simulink model "PF1_Q3"  (R2023b)
settings: Solver=FixedStepAuto  StartTime=0  StopTime=100  FixedStep=0.01  RelTol=1e-3
values from neighbouring files (symbols this model uses):
  B = double([diff(Xdot(1), u) ... (first row only)    [PF1.m]    (also in PF1_Q4.m)
  C = [1 0]    [PF1.m]    (also in PF1_Q4.m)
  K = place(A2, B, lambda_cl)    [PF1.m]    (also in PF1_Q4.m)
  K2 = place(A3, B, lambda_cl)    [PF1.m]    (also in PF1_Q4.m)
  Ki = -10    [PF1.m]    (also in PF1_Q4.m)
  xeq1 = double([eq.x1(1) ... (first row only)    [PF1.m]    (also in PF1_Q4.m = [0)
  xeq2 = double([eq.x1(2) ... (first row only)    [PF1.m]    (also in PF1_Q4.m = [1/2)
  xeq3 = [5 ... (first row only)    [PF1.m]    (also in PF1_Q4.m)
libraries: simulink x1
settings Model: Creator=therk  LastModifiedBy=Therkelsen

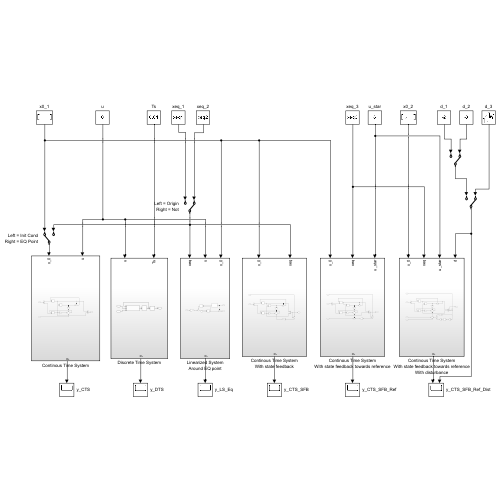
[thumbnail: Simulink's stored preview of the top-level diagram]
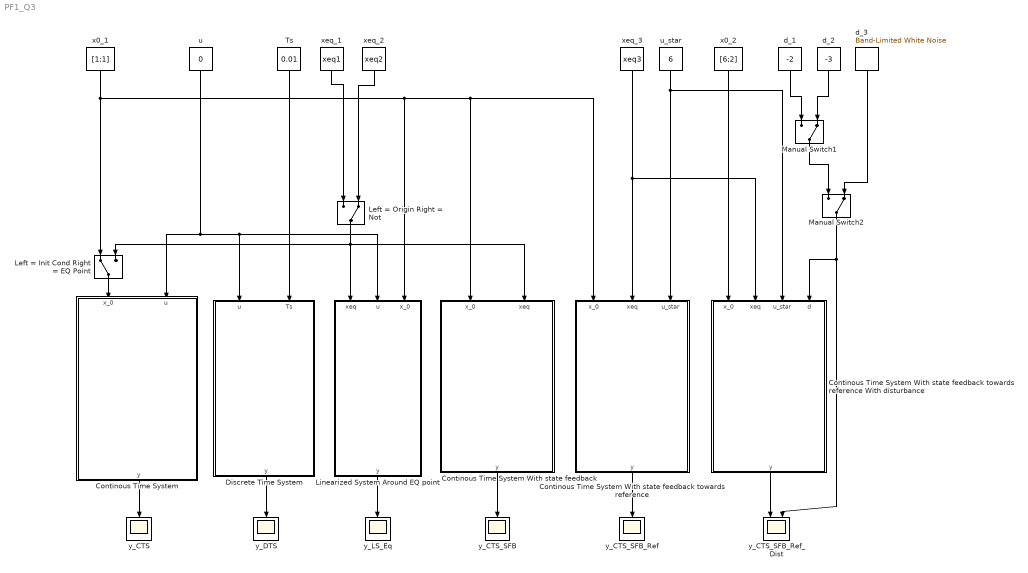
== system PF1_Q3 ==
  Continous Time System : Subsystem
  Continous Time System With state feedback : Subsystem
  Continous Time System With state feedback towards reference : Subsystem
  Continous Time System With state feedback towards reference With disturbance : Subsystem
  Discrete Time System : Subsystem
  Left = Init Cond Right = EQ Point : ManualSwitch
  Left = Origin Right = Not : ManualSwitch  CurrentSetting=0
  Linearized System Around EQ point : Subsystem
  Manual Switch1 : ManualSwitch  CurrentSetting=0
  Manual Switch2 : ManualSwitch  CurrentSetting=0
  Ts : Constant  Value=0.01
  d_1 : Constant  Value=-2
  d_2 : Constant  Value=-3
  d_3 : simulink/Sources/Band-Limited White Noise  Cov=[10]  Ts=10  seed=[23341]
  u : Constant  Value=0
  u_star : Constant  Value=6
  x0_1 : Constant  Value=[1;1]
  x0_2 : Constant  Value=[6;2]
  xeq_1 : Constant  Value=xeq1
  xeq_2 : Constant  Value=xeq2
  xeq_3 : Constant  Value=xeq3
  y_CTS : Scope
  y_CTS_SFB : Scope
  y_CTS_SFB_Ref : Scope
  y_CTS_SFB_Ref_Dist : Scope  NumInputPorts=2
  y_DTS : Scope
  y_LS_Eq : Scope
  wires:
  Continous Time System/1(y) -> y_CTS/1
  Ts/1 -> Discrete Time System/2(Ts)
  Discrete Time System/1(y) -> y_DTS/1
  xeq_2/1 -> Left = Origin Right = Not/2
  xeq_1/1 -> Left = Origin Right = Not/1
  Left = Origin Right = Not/1 -> Linearized System Around EQ point/1(xeq), Continous Time System With state feedback/2(xeq), Left = Init Cond Right = EQ Point/2
  u/1 -> Linearized System Around EQ point/2(u), Discrete Time System/1(u), Continous Time System/2(u)
  Linearized System Around EQ point/1(y) -> y_LS_Eq/1
  x0_1/1 -> Continous Time System With state feedback towards reference/1(x_0), Continous Time System With state feedback/1(x_0), Linearized System Around EQ point/3(x_0), Left = Init Cond Right = EQ Point/1
  Left = Init Cond Right = EQ Point/1 -> Continous Time System/1(x_0)
  Continous Time System With state feedback/1(y) -> y_CTS_SFB/1
  u_star/1 -> Continous Time System With state feedback towards reference With disturbance/3(u_star), Continous Time System With state feedback towards reference/3(u_star)
  Continous Time System With state feedback towards reference/1(y) -> y_CTS_SFB_Ref/1
  xeq_3/1 -> Continous Time System With state feedback towards reference With disturbance/2(xeq), Continous Time System With state feedback towards reference/2(xeq)
  Continous Time System With state feedback towards reference With disturbance/1(y) -> y_CTS_SFB_Ref_Dist/1
  d_1/1 -> Manual Switch1/1
  d_2/1 -> Manual Switch1/2
  x0_2/1 -> Continous Time System With state feedback towards reference With disturbance/1(x_0)
  d_3/1 -> Manual Switch2/2
  Manual Switch1/1 -> Manual Switch2/1
  Manual Switch2/1 -> y_CTS_SFB_Ref_Dist/2, Continous Time System With state feedback towards reference With disturbance/4(d)

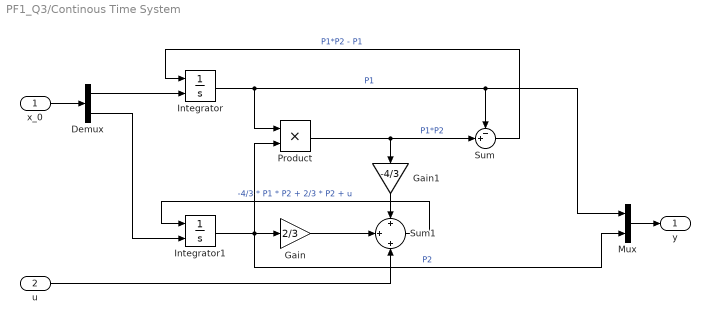
== system PF1_Q3/Continous Time System ==
  x_0 : Inport
  u : Inport  Port=2
  Demux : Demux  Outputs=2
  Gain : Gain  Gain=2/3
  Gain1 : Gain  Gain=-4/3
  Integrator : Integrator  InitialConditionSource=external
  Integrator1 : Integrator  InitialConditionSource=external
  Mux : Mux  Inputs=2
  Product : Product
  Sum : Sum  Inputs=-+|
  Sum1 : Sum  Inputs=+|+|+
  y : Outport
  wires:
  Gain1/1 -> Sum1/1
  Gain/1 -> Sum1/2
  u/1 -> Sum1/3
  Sum/1 -> Integrator/1  "P1*P2 - P1"
  Sum1/1 -> Integrator1/1  "-4/3 * P1 * P2 + 2/3 * P2 + u"
  Product/1 -> Sum/2, Gain1/1  "P1*P2"
  x_0/1 -> Demux/1
  Integrator/1 -> Mux/1, Sum/1, Product/1  "P1"
  Integrator1/1 -> Gain/1, Mux/2, Product/2  "P2"
  Mux/1 -> y/1
  Demux/2 -> Integrator1/2
  Demux/1 -> Integrator/2

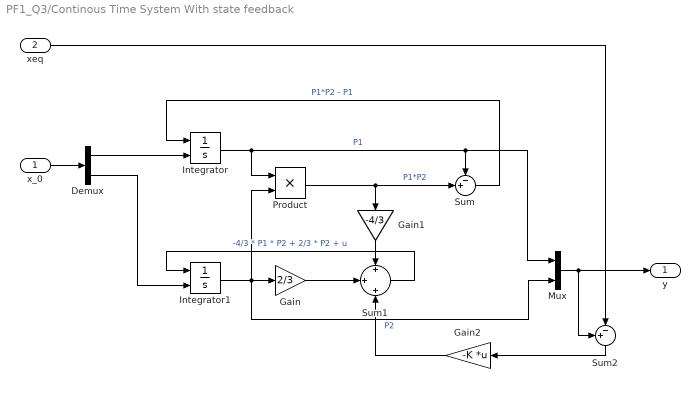
== system PF1_Q3/Continous Time System With state feedback ==
  x_0 : Inport
  xeq : Inport  Port=2
  Demux : Demux  Outputs=2
  Gain : Gain  Gain=2/3
  Gain1 : Gain  Gain=-4/3
  Gain2 : Gain  Gain=-K  Multiplication=Matrix(K*u)
  Integrator : Integrator  InitialConditionSource=external
  Integrator1 : Integrator  InitialConditionSource=external
  Mux : Mux  Inputs=2
  Product : Product
  Sum : Sum  Inputs=-+|
  Sum1 : Sum  Inputs=+|+|+
  Sum2 : Sum  Inputs=+-|
  y : Outport
  wires:
  Gain1/1 -> Sum1/1
  Gain/1 -> Sum1/2
  Sum/1 -> Integrator/1  "P1*P2 - P1"
  Sum1/1 -> Integrator1/1  "-4/3 * P1 * P2 + 2/3 * P2 + u"
  Product/1 -> Sum/2, Gain1/1  "P1*P2"
  x_0/1 -> Demux/1
  Integrator/1 -> Mux/1, Sum/1, Product/1  "P1"
  Integrator1/1 -> Mux/2, Gain/1, Product/2  "P2"
  Mux/1 -> y/1, Sum2/1
  Demux/2 -> Integrator1/2
  Demux/1 -> Integrator/2
  Sum2/1 -> Gain2/1
  xeq/1 -> Sum2/2
  Gain2/1 -> Sum1/3

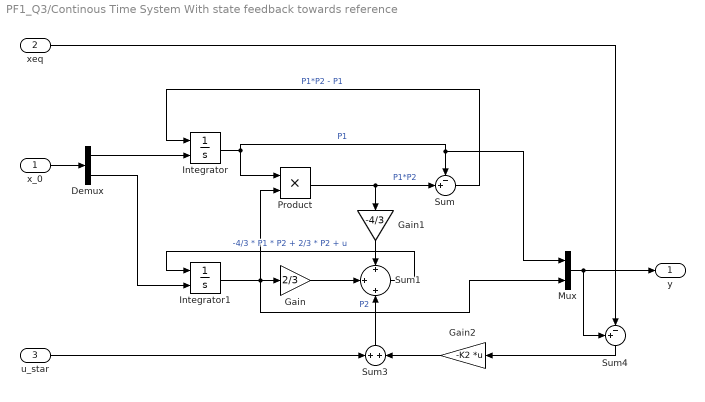
== system PF1_Q3/Continous Time System With state feedback towards reference ==
  x_0 : Inport
  xeq : Inport  Port=2
  u_star : Inport  Port=3
  Demux : Demux  Outputs=2
  Gain : Gain  Gain=2/3
  Gain1 : Gain  Gain=-4/3
  Gain2 : Gain  Gain=-K2  Multiplication=Matrix(K*u)
  Integrator : Integrator  InitialConditionSource=external
  Integrator1 : Integrator  InitialConditionSource=external
  Mux : Mux  Inputs=2
  Product : Product
  Sum : Sum  Inputs=-+|
  Sum1 : Sum  Inputs=+|+|+
  Sum3 : Sum  Inputs=+|+
  Sum4 : Sum  Inputs=+-|
  y : Outport
  wires:
  Gain1/1 -> Sum1/1
  Gain/1 -> Sum1/2
  Sum/1 -> Integrator/1  "P1*P2 - P1"
  Sum1/1 -> Integrator1/1  "-4/3 * P1 * P2 + 2/3 * P2 + u"
  Product/1 -> Sum/2, Gain1/1  "P1*P2"
  x_0/1 -> Demux/1
  Integrator/1 -> Mux/1, Sum/1, Product/1  "P1"
  Integrator1/1 -> Mux/2, Product/2, Gain/1  "P2"
  Mux/1 -> Sum4/1, y/1
  Demux/2 -> Integrator1/2
  Demux/1 -> Integrator/2
  xeq/1 -> Sum4/2
  Gain2/1 -> Sum3/2
  u_star/1 -> Sum3/1
  Sum3/1 -> Sum1/3
  Sum4/1 -> Gain2/1

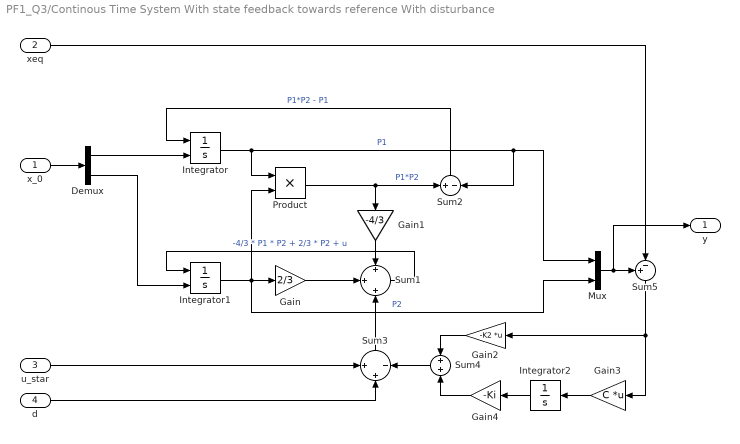
== system PF1_Q3/Continous Time System With state feedback towards reference With disturbance ==
  x_0 : Inport
  xeq : Inport  Port=2
  u_star : Inport  Port=3
  d : Inport  Port=4
  Demux : Demux  Outputs=2
  Gain : Gain  Gain=2/3
  Gain1 : Gain  Gain=-4/3
  Gain2 : Gain  Gain=-K2  Multiplication=Matrix(K*u)
  Gain3 : Gain  Gain=C  Multiplication=Matrix(K*u)
  Gain4 : Gain  Gain=-Ki
  Integrator : Integrator  InitialConditionSource=external
  Integrator1 : Integrator  InitialConditionSource=external
  Integrator2 : Integrator
  Mux : Mux  Inputs=2
  Product : Product
  Sum1 : Sum  Inputs=+|+|+
  Sum2 : Sum  Inputs=+|-
  Sum3 : Sum  Inputs=+|+|-
  Sum4 : Sum
  Sum5 : Sum  Inputs=+-|
  y : Outport
  wires:
  Gain1/1 -> Sum1/1
  Gain/1 -> Sum1/2
  Sum2/1 -> Integrator/1  "P1*P2 - P1"
  Sum1/1 -> Integrator1/1  "-4/3 * P1 * P2 + 2/3 * P2 + u"
  Product/1 -> Sum2/1, Gain1/1  "P1*P2"
  x_0/1 -> Demux/1
  Integrator/1 -> Sum2/2, Mux/1, Product/1  "P1"
  Integrator1/1 -> Mux/2, Gain/1, Product/2  "P2"
  Mux/1 -> Sum5/1, y/1
  Demux/2 -> Integrator1/2
  Demux/1 -> Integrator/2
  xeq/1 -> Sum5/2
  Gain2/1 -> Sum4/1
  u_star/1 -> Sum3/1
  Sum3/1 -> Sum1/3
  d/1 -> Sum3/2
  Gain3/1 -> Integrator2/1
  Integrator2/1 -> Gain4/1
  Gain4/1 -> Sum4/2
  Sum4/1 -> Sum3/3
  Sum5/1 -> Gain3/1, Gain2/1

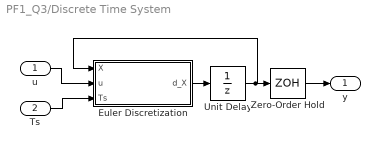
== system PF1_Q3/Discrete Time System ==
  u : Inport
  Ts : Inport  Port=2
  Euler Discretization : MATLAB Function  TreatAsAtomicUnit=on
  Unit Delay : UnitDelay  InitialCondition=[1;1]  SampleTime=-1  HasFrameUpgradeWarning=on
  Zero-Order Hold : ZeroOrderHold  SampleTime=-1
  y : Outport
  wires:
  Euler Discretization/1(d_X) -> Unit Delay/1
  Ts/1 -> Euler Discretization/3(Ts)
  Unit Delay/1 -> Zero-Order Hold/1, Euler Discretization/1(X)
  u/1 -> Euler Discretization/2(u)
  Zero-Order Hold/1 -> y/1

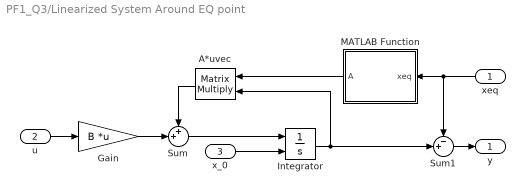
== system PF1_Q3/Linearized System Around EQ point ==
  xeq : Inport
  u : Inport  Port=2
  x_0 : Inport  Port=3
  A*uvec : Product  Multiplication=Matrix(*)
  Gain : Gain  Gain=B  Multiplication=Matrix(K*u) (u vector)
  Integrator : Integrator  InitialConditionSource=external  InitialCondition=[0.5;0]
  MATLAB Function : MATLAB Function  TreatAsAtomicUnit=on
  Sum : Sum  Inputs=++|
  Sum1 : Sum  Inputs=-+|
  y : Outport
  wires:
  u/1 -> Gain/1
  Integrator/1 -> Sum1/2, A*uvec/2
  x_0/1 -> Integrator/2
  Gain/1 -> Sum/2
  Sum/1 -> Integrator/1
  Sum1/1 -> y/1
  MATLAB Function/1(A) -> A*uvec/1
  A*uvec/1 -> Sum/1
  xeq/1 -> Sum1/1, MATLAB Function/1(xeq)

== matlab function PF1_Q3/Discrete Time System/Euler Discretization ==
  data: X input; d_X output; u input; Ts input
function d_X = fcn(X, u, Ts)

Xdot = [X(1)*X(2)-X(1);
        -4/3*X(1)*X(2)+2/3*X(2)+u];

d_X = [X(1) + Ts*Xdot(1);
          X(2) + Ts*Xdot(2)];

== matlab function PF1_Q3/Linearized System Around EQ point/MATLAB Function ==
  data: A output; xeq input
function A = fcn(xeq)
    A = computeA(xeq(1), xeq(2));
end
